simulink model "Series_Balancing"  (R2024b)
settings: Solver=FixedStepAuto  StartTime=0.0  StopTime=30  FixedStep=0.0001  RelTol=1e-3
model workspace (MAT data in the model file):
  Deg2Rad = 0.0174533
  Rad2Deg = 57.2957795
values from neighbouring files (symbols this model uses):
  D = zeros(6,2)    [old_Lqr_matrix.m]
  K = lqr(sys, Q, R)    [old_Lqr_matrix.m]
  X = [theta(t); theta_dot; x(t); x_dot; phi(t); phi_dot]    [old_Lqr_matrix.m]
undefined symbols (not defined in the file or in its folder): L0, Y, Z
libraries: sm_lib x47, nesl_utility x22, slpidlib x4
(part 3 of 3)

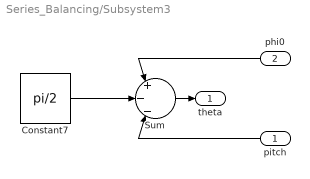
== system Series_Balancing/Subsystem3 ==
  pitch : Inport
  phi0 : Inport  Port=2
  Constant7 : Constant  Value=pi/2
  Sum : Sum  Inputs=|+|-|-|
  theta : Outport
  wires:
  Sum/1 -> theta/1
  Constant7/1 -> Sum/2
  pitch/1 -> Sum/3
  phi0/1 -> Sum/1

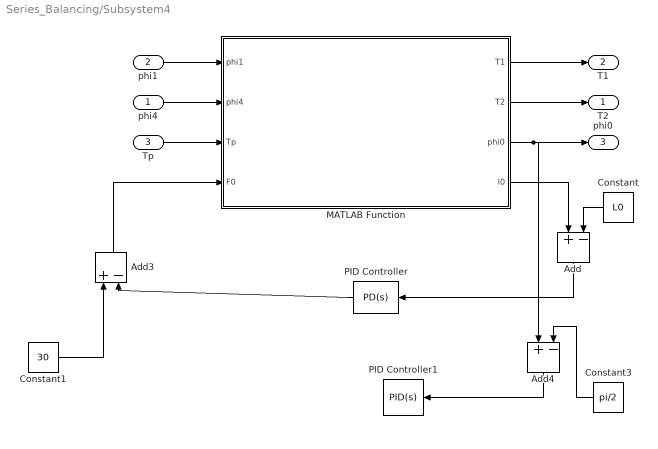
== system Series_Balancing/Subsystem4 ==
  phi4 : Inport
  phi1 : Inport  Port=2
  Tp : Inport  Port=3
  Add : Sum  Inputs=+|-
  Add3 : Sum  Inputs=+-
  Add4 : Sum  Inputs=+|-
  Constant : Constant  Value=L0
  Constant1 : Constant  Value=30
  Constant3 : Constant  Value=pi/2
  MATLAB Function : MATLAB Function  TreatAsAtomicUnit=on
  PID Controller : slpidlib/PID Controller  Controller=PD  Form=Parallel  TimeDomain=Continuous-time  UseExternalTs=off  SampleTime=-1  IntegratorMethod=Forward Euler  FilterMethod=Forward Euler  ControllerParametersSource=internal  P=3000  I=0  UseKiTs=off  D=200  UseExternalDerivativeSource=off  N=100  UseFilter=on  TunerSelectOption=Transfer Function Based (PID Tuner App)  InitialConditionSource=internal  InitialConditionForIntegrator=0  InitialConditionForFilter=0  DifferentiatorICPrevScaledInput=0  ExternalReset=none  TrackingMode=off  Kt=1  LimitOutput=on  SatLimitsSource=internal  UpperSaturationLimit=300  LowerSaturationLimit=-300  LinearizeAsGain=on  AntiWindupMode=none  Kb=1  LimitIntegrator=off  UpperIntegratorSaturationLimit=inf  LowerIntegratorSaturationLimit=-inf  POutMin=[]  POutMax=[]  IOutMin=[]  IOutMax=[]  DOutMin=[]  DOutMax=[]  NOutMin=[]  NOutMax=[]  SumOutMin=[]  SumOutMax=[]  SaturationOutMin=[]  SaturationOutMax=[]  PParamMin=[]  PParamMax=[]  IParamMin=[]  IParamMax=[]  DParamMin=[]  DParamMax=[]  NParamMin=[]  NParamMax=[]  KbParamMin=[]  KbParamMax=[]  KtParamMin=[]  KtParamMax=[]  KbOutMin=[]  KbOutMax=[]  KtOutMin=[]  KtOutMax=[]  IntegratorOutMin=[]  IntegratorOutMax=[]  FilterOutMin=[]  FilterOutMax=[]  SumI1OutMin=[]  SumI1OutMax=[]  SumI2OutMin=[]  SumI2OutMax=[]  SumI3OutMin=[]  SumI3OutMax=[]  SumI4OutMin=[]  SumI4OutMax=[]  SumDOutMin=[]  SumDOutMax=[]  DifferentiatorOutMin=[]  DifferentiatorOutMax=[]  FilterDiffOutCoefMin=[]  FilterDiffOutCoefMax=[]  ReciprocalOutMin=[]  ReciprocalOutMax=[]  SumDenOutMin=[]  SumDenOutMax=[]  SumNumOutMin=[]  SumNumOutMax=[]  DivideOutMin=[]  DivideOutMax=[]  UdiffTsProdOutMin=[]  UdiffTsProdOutMax=[]  NTsProdOutMin=[]  NTsProdOutMax=[]  UintegralTsProdOutMin=[]  UintegralTsProdOutMax=[]  UngainTsProdOutMin=[]  UngainTsProdOutMax=[]  ClampingZeroOutDataTypeStr=Inherit: Inherit via back propagation  ClampingZeroOutMin=[]  ClampingZeroOutMax=[]  FilterDenConstantOutDataTypeStr=Inherit: Inherit via back propagation  FilterDenConstantOutMin=[]  FilterDenConstantOutMax=[]  PCopyOutDataTypeStr=Inherit: Inherit via back propagation  PCopyOutMin=[]  PCopyOutMax=[]  NCopyOutDataTypeStr=Inherit: Inherit via back propagation  NCopyOutMin=[]  NCopyOutMax=[]  IntegratorContinuousStateAttributes=''  IntegratorStateMustResolveToSignalObject=off  IntegratorRTWStateStorageClass=Auto  FilterContinuousStateAttributes=''  FilterStateMustResolveToSignalObject=off  FilterRTWStateStorageClass=Auto  ParallelPVariant=InternalParameters  IdealPVariant=Disabled  IVariant=Disabled  DVariant=InternalParameters  IntegratorVariant=Disabled  SatVariant=Enabled  AWVariant=Disabled  PCopyVariant=Disabled  TRVariant=Disabled  FdbkBlocksVariant=Forward  IdealPFdbkVariant=Disabled  SatFdbkVariant=Disabled  DerivativeFilterVariant=ContFilter  NVariant=InternalParameters  NCopyVariant=Disabled  FilterICVariant=InternalICsFilter  IntegratorICVariant=Disabled  ExternalResetVariant=Disabled  TRSumVariant=Passthrough  SumFdbkVariant=Disabled  SumVariant=Sum_PD  TsampFilterVariant=InternalTs  TsampNgainVariant=Passthrough  TsampIntegralVariant=Disabled_SignalSpec  ExternalSaturationOutDataTypeStr=Inherit: Same as second input  DerivativeSourceVariant=ErrorSignal  PreIntVariant=InternalPreInt
  PID Controller1 : slpidlib/PID Controller  Controller=PID  Form=Parallel  TimeDomain=Continuous-time  UseExternalTs=off  SampleTime=-1  IntegratorMethod=Forward Euler  FilterMethod=Forward Euler  ControllerParametersSource=internal  P=100  I=0  UseKiTs=off  D=1  UseExternalDerivativeSource=off  N=100  UseFilter=on  TunerSelectOption=Transfer Function Based (PID Tuner App)  InitialConditionSource=internal  InitialConditionForIntegrator=0  InitialConditionForFilter=0  DifferentiatorICPrevScaledInput=0  ExternalReset=none  TrackingMode=off  Kt=1  LimitOutput=off  SatLimitsSource=internal  UpperSaturationLimit=inf  LowerSaturationLimit=-inf  LinearizeAsGain=on  AntiWindupMode=none  Kb=1  LimitIntegrator=off  UpperIntegratorSaturationLimit=inf  LowerIntegratorSaturationLimit=-inf  POutMin=[]  POutMax=[]  IOutMin=[]  IOutMax=[]  DOutMin=[]  DOutMax=[]  NOutMin=[]  NOutMax=[]  SumOutMin=[]  SumOutMax=[]  SaturationOutMin=[]  SaturationOutMax=[]  PParamMin=[]  PParamMax=[]  IParamMin=[]  IParamMax=[]  DParamMin=[]  DParamMax=[]  NParamMin=[]  NParamMax=[]  KbParamMin=[]  KbParamMax=[]  KtParamMin=[]  KtParamMax=[]  KbOutMin=[]  KbOutMax=[]  KtOutMin=[]  KtOutMax=[]  IntegratorOutMin=[]  IntegratorOutMax=[]  FilterOutMin=[]  FilterOutMax=[]  SumI1OutMin=[]  SumI1OutMax=[]  SumI2OutMin=[]  SumI2OutMax=[]  SumI3OutMin=[]  SumI3OutMax=[]  SumI4OutMin=[]  SumI4OutMax=[]  SumDOutMin=[]  SumDOutMax=[]  DifferentiatorOutMin=[]  DifferentiatorOutMax=[]  FilterDiffOutCoefMin=[]  FilterDiffOutCoefMax=[]  ReciprocalOutMin=[]  ReciprocalOutMax=[]  SumDenOutMin=[]  SumDenOutMax=[]  SumNumOutMin=[]  SumNumOutMax=[]  DivideOutMin=[]  DivideOutMax=[]  UdiffTsProdOutMin=[]  UdiffTsProdOutMax=[]  NTsProdOutMin=[]  NTsProdOutMax=[]  UintegralTsProdOutMin=[]  UintegralTsProdOutMax=[]  UngainTsProdOutMin=[]  UngainTsProdOutMax=[]  ClampingZeroOutDataTypeStr=Inherit: Inherit via back propagation  ClampingZeroOutMin=[]  ClampingZeroOutMax=[]  FilterDenConstantOutDataTypeStr=Inherit: Inherit via back propagation  FilterDenConstantOutMin=[]  FilterDenConstantOutMax=[]  PCopyOutDataTypeStr=Inherit: Inherit via back propagation  PCopyOutMin=[]  PCopyOutMax=[]  NCopyOutDataTypeStr=Inherit: Inherit via back propagation  NCopyOutMin=[]  NCopyOutMax=[]  IntegratorContinuousStateAttributes=''  IntegratorStateMustResolveToSignalObject=off  IntegratorRTWStateStorageClass=Auto  FilterContinuousStateAttributes=''  FilterStateMustResolveToSignalObject=off  FilterRTWStateStorageClass=Auto  ParallelPVariant=InternalParameters  IdealPVariant=Disabled  IVariant=InternalParameters  DVariant=InternalParameters  IntegratorVariant=Continuous  SatVariant=Disabled  AWVariant=Passthrough  PCopyVariant=Disabled  TRVariant=Disabled  FdbkBlocksVariant=Forward  IdealPFdbkVariant=Disabled  SatFdbkVariant=Disabled  DerivativeFilterVariant=ContFilter  NVariant=InternalParameters  NCopyVariant=Disabled  FilterICVariant=InternalICsFilter  IntegratorICVariant=InternalICs  ExternalResetVariant=Disabled  TRSumVariant=Passthrough  SumFdbkVariant=Disabled  SumVariant=Sum_PID  TsampFilterVariant=InternalTs  TsampNgainVariant=Passthrough  TsampIntegralVariant=Disabled_SignalSpec  ExternalSaturationOutDataTypeStr=Inherit: Same as second input  DerivativeSourceVariant=ErrorSignal  PreIntVariant=InternalPreInt
  T2 : Outport
  T1 : Outport  Port=2
  phi0 : Outport  Port=3
  wires:
  PID Controller/1 -> Add3/2
  Add3/1 -> MATLAB Function/4(F0)
  MATLAB Function/1(T1) -> T1/1
  MATLAB Function/2(T2) -> T2/1
  MATLAB Function/4(l0) -> Add/1
  Constant3/1 -> Add4/2
  phi1/1 -> MATLAB Function/1(phi1)
  MATLAB Function/3(phi0) -> Add4/1, phi0/1
  phi4/1 -> MATLAB Function/2(phi4)
  Add4/1 -> PID Controller1/1
  Constant/1 -> Add/2
  Constant1/1 -> Add3/1
  Add/1 -> PID Controller/1
  Tp/1 -> MATLAB Function/3(Tp)

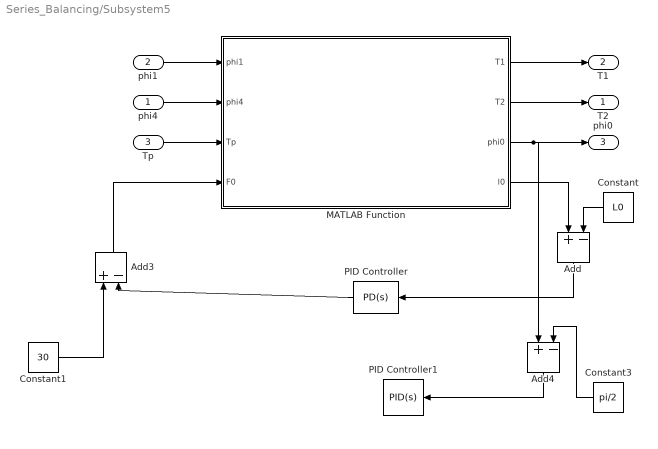
== system Series_Balancing/Subsystem5 ==
  phi4 : Inport
  phi1 : Inport  Port=2
  Tp : Inport  Port=3
  Add : Sum  Inputs=+|-
  Add3 : Sum  Inputs=+-
  Add4 : Sum  Inputs=+|-
  Constant : Constant  Value=L0
  Constant1 : Constant  Value=30
  Constant3 : Constant  Value=pi/2
  MATLAB Function : MATLAB Function  TreatAsAtomicUnit=on
  PID Controller : slpidlib/PID Controller  Controller=PD  Form=Parallel  TimeDomain=Continuous-time  UseExternalTs=off  SampleTime=-1  IntegratorMethod=Forward Euler  FilterMethod=Forward Euler  ControllerParametersSource=internal  P=3000  I=0  UseKiTs=off  D=120  UseExternalDerivativeSource=off  N=100  UseFilter=on  TunerSelectOption=Transfer Function Based (PID Tuner App)  InitialConditionSource=internal  InitialConditionForIntegrator=0  InitialConditionForFilter=0  DifferentiatorICPrevScaledInput=0  ExternalReset=none  TrackingMode=off  Kt=1  LimitOutput=on  SatLimitsSource=internal  UpperSaturationLimit=300  LowerSaturationLimit=-300  LinearizeAsGain=on  AntiWindupMode=none  Kb=1  LimitIntegrator=off  UpperIntegratorSaturationLimit=inf  LowerIntegratorSaturationLimit=-inf  POutMin=[]  POutMax=[]  IOutMin=[]  IOutMax=[]  DOutMin=[]  DOutMax=[]  NOutMin=[]  NOutMax=[]  SumOutMin=[]  SumOutMax=[]  SaturationOutMin=[]  SaturationOutMax=[]  PParamMin=[]  PParamMax=[]  IParamMin=[]  IParamMax=[]  DParamMin=[]  DParamMax=[]  NParamMin=[]  NParamMax=[]  KbParamMin=[]  KbParamMax=[]  KtParamMin=[]  KtParamMax=[]  KbOutMin=[]  KbOutMax=[]  KtOutMin=[]  KtOutMax=[]  IntegratorOutMin=[]  IntegratorOutMax=[]  FilterOutMin=[]  FilterOutMax=[]  SumI1OutMin=[]  SumI1OutMax=[]  SumI2OutMin=[]  SumI2OutMax=[]  SumI3OutMin=[]  SumI3OutMax=[]  SumI4OutMin=[]  SumI4OutMax=[]  SumDOutMin=[]  SumDOutMax=[]  DifferentiatorOutMin=[]  DifferentiatorOutMax=[]  FilterDiffOutCoefMin=[]  FilterDiffOutCoefMax=[]  ReciprocalOutMin=[]  ReciprocalOutMax=[]  SumDenOutMin=[]  SumDenOutMax=[]  SumNumOutMin=[]  SumNumOutMax=[]  DivideOutMin=[]  DivideOutMax=[]  UdiffTsProdOutMin=[]  UdiffTsProdOutMax=[]  NTsProdOutMin=[]  NTsProdOutMax=[]  UintegralTsProdOutMin=[]  UintegralTsProdOutMax=[]  UngainTsProdOutMin=[]  UngainTsProdOutMax=[]  ClampingZeroOutDataTypeStr=Inherit: Inherit via back propagation  ClampingZeroOutMin=[]  ClampingZeroOutMax=[]  FilterDenConstantOutDataTypeStr=Inherit: Inherit via back propagation  FilterDenConstantOutMin=[]  FilterDenConstantOutMax=[]  PCopyOutDataTypeStr=Inherit: Inherit via back propagation  PCopyOutMin=[]  PCopyOutMax=[]  NCopyOutDataTypeStr=Inherit: Inherit via back propagation  NCopyOutMin=[]  NCopyOutMax=[]  IntegratorContinuousStateAttributes=''  IntegratorStateMustResolveToSignalObject=off  IntegratorRTWStateStorageClass=Auto  FilterContinuousStateAttributes=''  FilterStateMustResolveToSignalObject=off  FilterRTWStateStorageClass=Auto  ParallelPVariant=InternalParameters  IdealPVariant=Disabled  IVariant=Disabled  DVariant=InternalParameters  IntegratorVariant=Disabled  SatVariant=Enabled  AWVariant=Disabled  PCopyVariant=Disabled  TRVariant=Disabled  FdbkBlocksVariant=Forward  IdealPFdbkVariant=Disabled  SatFdbkVariant=Disabled  DerivativeFilterVariant=ContFilter  NVariant=InternalParameters  NCopyVariant=Disabled  FilterICVariant=InternalICsFilter  IntegratorICVariant=Disabled  ExternalResetVariant=Disabled  TRSumVariant=Passthrough  SumFdbkVariant=Disabled  SumVariant=Sum_PD  TsampFilterVariant=InternalTs  TsampNgainVariant=Passthrough  TsampIntegralVariant=Disabled_SignalSpec  ExternalSaturationOutDataTypeStr=Inherit: Same as second input  DerivativeSourceVariant=ErrorSignal  PreIntVariant=InternalPreInt
  PID Controller1 : slpidlib/PID Controller  Controller=PID  Form=Parallel  TimeDomain=Continuous-time  UseExternalTs=off  SampleTime=-1  IntegratorMethod=Forward Euler  FilterMethod=Forward Euler  ControllerParametersSource=internal  P=100  I=0  UseKiTs=off  D=1  UseExternalDerivativeSource=off  N=100  UseFilter=on  TunerSelectOption=Transfer Function Based (PID Tuner App)  InitialConditionSource=internal  InitialConditionForIntegrator=0  InitialConditionForFilter=0  DifferentiatorICPrevScaledInput=0  ExternalReset=none  TrackingMode=off  Kt=1  LimitOutput=off  SatLimitsSource=internal  UpperSaturationLimit=inf  LowerSaturationLimit=-inf  LinearizeAsGain=on  AntiWindupMode=none  Kb=1  LimitIntegrator=off  UpperIntegratorSaturationLimit=inf  LowerIntegratorSaturationLimit=-inf  POutMin=[]  POutMax=[]  IOutMin=[]  IOutMax=[]  DOutMin=[]  DOutMax=[]  NOutMin=[]  NOutMax=[]  SumOutMin=[]  SumOutMax=[]  SaturationOutMin=[]  SaturationOutMax=[]  PParamMin=[]  PParamMax=[]  IParamMin=[]  IParamMax=[]  DParamMin=[]  DParamMax=[]  NParamMin=[]  NParamMax=[]  KbParamMin=[]  KbParamMax=[]  KtParamMin=[]  KtParamMax=[]  KbOutMin=[]  KbOutMax=[]  KtOutMin=[]  KtOutMax=[]  IntegratorOutMin=[]  IntegratorOutMax=[]  FilterOutMin=[]  FilterOutMax=[]  SumI1OutMin=[]  SumI1OutMax=[]  SumI2OutMin=[]  SumI2OutMax=[]  SumI3OutMin=[]  SumI3OutMax=[]  SumI4OutMin=[]  SumI4OutMax=[]  SumDOutMin=[]  SumDOutMax=[]  DifferentiatorOutMin=[]  DifferentiatorOutMax=[]  FilterDiffOutCoefMin=[]  FilterDiffOutCoefMax=[]  ReciprocalOutMin=[]  ReciprocalOutMax=[]  SumDenOutMin=[]  SumDenOutMax=[]  SumNumOutMin=[]  SumNumOutMax=[]  DivideOutMin=[]  DivideOutMax=[]  UdiffTsProdOutMin=[]  UdiffTsProdOutMax=[]  NTsProdOutMin=[]  NTsProdOutMax=[]  UintegralTsProdOutMin=[]  UintegralTsProdOutMax=[]  UngainTsProdOutMin=[]  UngainTsProdOutMax=[]  ClampingZeroOutDataTypeStr=Inherit: Inherit via back propagation  ClampingZeroOutMin=[]  ClampingZeroOutMax=[]  FilterDenConstantOutDataTypeStr=Inherit: Inherit via back propagation  FilterDenConstantOutMin=[]  FilterDenConstantOutMax=[]  PCopyOutDataTypeStr=Inherit: Inherit via back propagation  PCopyOutMin=[]  PCopyOutMax=[]  NCopyOutDataTypeStr=Inherit: Inherit via back propagation  NCopyOutMin=[]  NCopyOutMax=[]  IntegratorContinuousStateAttributes=''  IntegratorStateMustResolveToSignalObject=off  IntegratorRTWStateStorageClass=Auto  FilterContinuousStateAttributes=''  FilterStateMustResolveToSignalObject=off  FilterRTWStateStorageClass=Auto  ParallelPVariant=InternalParameters  IdealPVariant=Disabled  IVariant=InternalParameters  DVariant=InternalParameters  IntegratorVariant=Continuous  SatVariant=Disabled  AWVariant=Passthrough  PCopyVariant=Disabled  TRVariant=Disabled  FdbkBlocksVariant=Forward  IdealPFdbkVariant=Disabled  SatFdbkVariant=Disabled  DerivativeFilterVariant=ContFilter  NVariant=InternalParameters  NCopyVariant=Disabled  FilterICVariant=InternalICsFilter  IntegratorICVariant=InternalICs  ExternalResetVariant=Disabled  TRSumVariant=Passthrough  SumFdbkVariant=Disabled  SumVariant=Sum_PID  TsampFilterVariant=InternalTs  TsampNgainVariant=Passthrough  TsampIntegralVariant=Disabled_SignalSpec  ExternalSaturationOutDataTypeStr=Inherit: Same as second input  DerivativeSourceVariant=ErrorSignal  PreIntVariant=InternalPreInt
  T2 : Outport
  T1 : Outport  Port=2
  phi0 : Outport  Port=3
  wires:
  MATLAB Function/3(phi0) -> Add4/1, phi0/1
  Constant3/1 -> Add4/2
  Add/1 -> PID Controller/1
  Constant/1 -> Add/2
  Add4/1 -> PID Controller1/1
  MATLAB Function/4(l0) -> Add/1
  phi1/1 -> MATLAB Function/1(phi1)
  phi4/1 -> MATLAB Function/2(phi4)
  MATLAB Function/1(T1) -> T1/1
  MATLAB Function/2(T2) -> T2/1
  Constant1/1 -> Add3/1
  Add3/1 -> MATLAB Function/4(F0)
  PID Controller/1 -> Add3/2
  Tp/1 -> MATLAB Function/3(Tp)

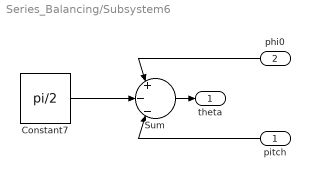
== system Series_Balancing/Subsystem6 ==
  pitch : Inport
  phi0 : Inport  Port=2
  Constant7 : Constant  Value=pi/2
  Sum : Sum  Inputs=|+|-|-|
  theta : Outport
  wires:
  Sum/1 -> theta/1
  Constant7/1 -> Sum/2
  pitch/1 -> Sum/3
  phi0/1 -> Sum/1

== matlab function Series_Balancing/MATLAB Function ==
  data: phi1 input; d_phi0 output; phi4 input; d_phi1 input; d_phi4 input
function d_phi0 = d_phi0_cal(phi1,phi4,d_phi1,d_phi4)
K1 = 2.1875;
l1 = 0.08;
l2 = 0.08;
l3 = 0.08;
l4 = 0.08;
Xb = l1 * cos(phi1);
Yb = l1 * sin(phi1);
Xd = l4 * cos(phi4);
Yd = l4 * sin(phi4);

Lbd2 = (Xd - Xb)*(Xd - Xb) + (Yd - Yb)*(Xd - Xb);
a = 2*l2* (Xd - Xb);
b = 2*l2* (Yd - Yb);
c = l2*l2 - l3*l3 + Lbd2;
phi2 = phi4;
phi3 = phi1;
% phi2 = 2*atan2((b + sqrt(a*a + b*b - c*c)),(a + c));
% phi3 = atan2(Yb-Yd+l2*sin(phi2),Xb-Xd+l2*cos(phi2));
Xc = Xb + l2*cos(phi2);
Yc = Yb + l2*sin(phi2);
% Xf = K1*Xc;
% Yf = K1*Yc;
phi_dot_1 = d_phi1;
phi_dot_4 = d_phi4;
d_phi0 = ((l1*phi_dot_1*cos(phi1) + l2*phi_dot_4*cos(phi4))/(l1*cos(phi1) + l2*cos(phi4)) + ((l1*phi_dot_1*sin(phi1) + l2*phi_dot_4*sin(phi4))*(l1*sin(phi1) + l2*sin(phi4)))/(l1*cos(phi1) + l2*cos(phi4))^2)/((l1*sin(phi1) + l2*sin(phi4))^2/(l1*cos(phi1) + l2*cos(phi4))^2 + 1);

end

== matlab function Series_Balancing/Subsystem4/MATLAB Function ==
  data: phi1 input; T1 output; phi4 input; T2 output; Tp input; F0 input; phi0 output; l0 output
function [T1,T2,phi0,l0] = VMC(phi1 , phi4 , Tp , F0)
K1 = 2.1875;
l1 = 0.08;
l2 = 0.08;
l3 = 0.08;
l4 = 0.08;
Xb = l1 * cos(phi1);
Yb = l1 * sin(phi1);
Xd = l4 * cos(phi4);
Yd = l4 * sin(phi4);

Lbd2 = (Xd - Xb)*(Xd - Xb) + (Yd - Yb)*(Yd - Yb);
a = 2*l2* (Xd - Xb);
b = 2*l2* (Yd - Yb);
c = l2*l2 - l3*l3 + Lbd2;
% phi2 = phi4;
% phi3 = phi1;
phi2 = 2*atan2((b + sqrt(a*a + b*b - c*c)),(a + c));
phi3 = atan2(Yb-Yd+l2*sin(phi2),Xb-Xd+l2*cos(phi2));
Xc = Xb + l2*cos(phi2);
Yc = Yb + l2*sin(phi2);
Xf = K1*Xc;
Yf = K1*Yc;
phi0 = atan2(Yf,Xf);
l0 = sqrt(Xf*Xf + Yf*Yf);

J11 = -(K1*l1*sin(phi0 - phi3)*sin(phi1 - phi2))/sin(phi2 - phi3);
J12 = -(K1*l1*cos(phi0 - phi3)*sin(phi1 - phi2))/(l0*sin(phi2 - phi3));
J21 = -(K1*l4*sin(phi0 - phi2)*sin(phi3 - phi4))/sin(phi2 - phi3);
J22 = -(K1*l4*cos(phi0 - phi2)*sin(phi3 - phi4))/(l0*sin(phi2 - phi3));

J = [J11 J12;
     J21 J22];
F = [F0 ; Tp];
T = J*F;
T1 = T(1,1);
T2 = T(2,1);
end

== matlab function Series_Balancing/MATLAB Function2 ==
  data: q input; yaw output; pitch output; roll output
function [yaw,pitch,roll] = QuatToEuler(q)
%#codegen
% q: quaternion [qw qx qy qz]
% eul: [yaw pitch roll] in radians, ZYX rotation sequence

% 确保是列向量
q = q(:);
qw = q(1);
qx = q(2);
qy = q(3);
qz = q(4);

% --- 计算旋转矩阵 ---
R = [1 - 2*(qy^2 + qz^2),     2*(qx*qy - qz*qw),     2*(qx*qz + qy*qw);
     2*(qx*qy + qz*qw),       1 - 2*(qx^2 + qz^2),   2*(qy*qz - qx*qw);
     2*(qx*qz - qy*qw),       2*(qy*qz + qx*qw),     1 - 2*(qx^2 + qy^2)];

% --- 提取欧拉角（ZYX顺序） ---
yaw   = atan2(R(2,1), R(1,1));       % 绕Z轴
pitch = asin(-R(3,1));               % 绕Y轴
roll  = atan2(R(3,2), R(3,3));       % 绕X轴

== matlab function Series_Balancing/Subsystem5/MATLAB Function ==
  data: phi1 input; T1 output; phi4 input; T2 output; Tp input; F0 input; phi0 output; l0 output
function [T1,T2,phi0,l0] = VMC(phi1 , phi4 , Tp , F0)
K1 = 2.1875;
l1 = 0.08;
l2 = 0.08;
l3 = 0.08;
l4 = 0.08;
Xb = l1 * cos(phi1);
Yb = l1 * sin(phi1);
Xd = l4 * cos(phi4);
Yd = l4 * sin(phi4);

Lbd2 = (Xd - Xb)*(Xd - Xb) + (Yd - Yb)*(Yd - Yb);
a = 2*l2* (Xd - Xb);
b = 2*l2* (Yd - Yb);
c = l2*l2 - l3*l3 + Lbd2;
% phi2 = phi4;
% phi3 = phi1;
phi2 = 2*atan2((b + sqrt(a*a + b*b - c*c)),(a + c));
phi3 = atan2(Yb-Yd+l2*sin(phi2),Xb-Xd+l2*cos(phi2));
Xc = Xb + l2*cos(phi2);
Yc = Yb + l2*sin(phi2);
Xf = K1*Xc;
Yf = K1*Yc;
phi0 = atan2(Yf,Xf);
l0 = sqrt(Xf*Xf + Yf*Yf);

J11 = -(K1*l1*sin(phi0 - phi3)*sin(phi1 - phi2))/sin(phi2 - phi3);
J12 = -(K1*l1*cos(phi0 - phi3)*sin(phi1 - phi2))/(l0*sin(phi2 - phi3));
J21 = -(K1*l4*sin(phi0 - phi2)*sin(phi3 - phi4))/sin(phi2 - phi3);
J22 = -(K1*l4*cos(phi0 - phi2)*sin(phi3 - phi4))/(l0*sin(phi2 - phi3));

J = [J11 J12;
     J21 J22];
F = [F0 ; Tp];
T = J*F;
T1 = T(1,1);
T2 = T(2,1);
end

== matlab function Series_Balancing/MATLAB Function1 ==
  data: phi1 input; d_phi0 output; phi4 input; d_phi1 input; d_phi4 input
function d_phi0 = d_phi0_cal(phi1,phi4,d_phi1,d_phi4)
K1 = 2.1875;
l1 = 0.08;
l2 = 0.08;
l3 = 0.08;
l4 = 0.08;
Xb = l1 * cos(phi1);
Yb = l1 * sin(phi1);
Xd = l4 * cos(phi4);
Yd = l4 * sin(phi4);

Lbd2 = (Xd - Xb)*(Xd - Xb) + (Yd - Yb)*(Xd - Xb);
a = 2*l2* (Xd - Xb);
b = 2*l2* (Yd - Yb);
c = l2*l2 - l3*l3 + Lbd2;
phi2 = phi4;
phi3 = phi1;
% phi2 = 2*atan2((b + sqrt(a*a + b*b - c*c)),(a + c));
% phi3 = atan2(Yb-Yd+l2*sin(phi2),Xb-Xd+l2*cos(phi2));
Xc = Xb + l2*cos(phi2);
Yc = Yb + l2*sin(phi2);
% Xf = K1*Xc;
% Yf = K1*Yc;
phi_dot_1 = d_phi1;
phi_dot_4 = d_phi4;
d_phi0 = ((l1*phi_dot_1*cos(phi1) + l2*phi_dot_4*cos(phi4))/(l1*cos(phi1) + l2*cos(phi4)) + ((l1*phi_dot_1*sin(phi1) + l2*phi_dot_4*sin(phi4))*(l1*sin(phi1) + l2*sin(phi4)))/(l1*cos(phi1) + l2*cos(phi4))^2)/((l1*sin(phi1) + l2*sin(phi4))^2/(l1*cos(phi1) + l2*cos(phi4))^2 + 1);

end

== matlab function Series_Balancing/Subsystem/MATLAB Function ==
  data: u input; t output; tp output; K input
function [t,tp] = lqr_outputCal(u,K)
T = -K * u;
t = T(1);
tp = T(2);
end

== matlab function Series_Balancing/Subsystem1/MATLAB Function ==
  data: u input; t output; tp output; K input
function [t,tp] = lqr_outputCal(u,K)
T = -K * u;
t = T(1);
tp = T(2);
end
